simulink model "disturbance_est"  (R2020b)
settings: Solver=FixedStepAuto  StartTime=0.0  StopTime=10  FixedStep=0.01  RelTol=1e-3
values from neighbouring files (symbols this model uses):
  G = -J_RH*(M_M*L/2+M*l)*(J_RH+N^2*J_m+j)*g    (= -0.22537747671)    [aaaaaaaaaaaaaaaaaaaaaaaaa.m]    (also in disturb_estimation.m = -0.0465293382657; full_obs2.m = -0.0465293382657; fuulll_feedback.m = -0.0465293382657; reduced_observre_2.m = -0.0465293382657)
  H = -N*K_m*J_RH    (= -0.00759948)    [aaaaaaaaaaaaaaaaaaaaaaaaa.m]    (also in disturb_estimation.m = -0.00486576; full_obs2.m = -0.00486576; fuulll_feedback.m = -0.00486576; reduced_observre_2.m = -0.00486576)
  k1 = K(1)    [disturb_estimation.m]    (also in full_obs2.m; fuulll_feedback.m; reduced_observre_2.m)
  k2 = K(2)    [disturb_estimation.m]    (also in full_obs2.m; fuulll_feedback.m; reduced_observre_2.m)
  k3 = K(3)    [disturb_estimation.m]    (also in full_obs2.m; fuulll_feedback.m; reduced_observre_2.m)
  k4 = K(4)    [disturb_estimation.m]    (also in full_obs2.m; fuulll_feedback.m; reduced_observre_2.m)
  k5 = K(5)    [disturb_estimation.m]    (also in full_obs2.m; fuulll_feedback.m; reduced_observre_2.m)
  K_m = 0.0109    [aaaaaaaaaaaaaaaaaaaaaaaaa.m]    (also in disturb_estimation.m; full_obs2.m; fuulll_feedback.m; reduced_observre_2.m)
  l1 = L(1)    [disturb_estimation.m]    (also in full (2).m = 0.06; full_obs2.m)
  l2 = L(2)    [disturb_estimation.m]    (also in full (2).m = 0.6329; full_obs2.m)
  l3 = L(3)    [disturb_estimation.m]    (also in full (2).m = 0.3; full_obs2.m)
  l4 = L(4)    [disturb_estimation.m]    (also in full (2).m = 0.0875; full_obs2.m)
  l5 = L(5)    [disturb_estimation.m]    (also in full (2).m = 0.0254; full_obs2.m)
  l6 = 160    [disturb_estimation.m]    (also in full_obs2.m = 100)
  L_m = 0.145    [aaaaaaaaaaaaaaaaaaaaaaaaa.m]    (also in disturb_estimation.m; full_obs2.m; fuulll_feedback.m; reduced_observre_2.m)
  N = 14    [aaaaaaaaaaaaaaaaaaaaaaaaa.m]    (also in disturb_estimation.m = 3; full (2).m = -1.06605676; full_obs2.m = 3; fuulll_feedback.m = 3)
  R_m = 1.6    [aaaaaaaaaaaaaaaaaaaaaaaaa.m]    (also in disturb_estimation.m; full_obs2.m; fuulll_feedback.m; reduced_observre_2.m)
  T = (M_M*L/2+M*l)*(J_RH+N^2*J_m+j)*g    (= 4.52565214276)    [aaaaaaaaaaaaaaaaaaaaaaaaa.m]    (also in disturb_estimation.m = 0.312697165764; full (2).m = [T1;T2;T3;T4;T5;T6;T7]; full_obs2.m = 0.312697165764; fuulll_feedback.m = 0.312697165764)
  W = (J_M+M*l^2)*(J_RH+N^2*J_m+j)-(J_RH)^2    (= 0.0397505665657)    [aaaaaaaaaaaaaaaaaaaaaaaaa.m]    (also in disturb_estimation.m = -0.0192235420783; full (2).m = blkdiag(W_1,W_2,W_3,W_4,W_5,W_6,W_7); full_obs2.m = -0.0192235420783; fuulll_feedback.m = -0.0192235420783)
  Z = (J_M+M*l^2)*(J_RH+N^2*J_m+j)^2-J_RH^2*(J_RH+N^2*J_m+j)    (= 0.251295170273)    [aaaaaaaaaaaaaaaaaaaaaaaaa.m]    (also in disturb_estimation.m = -0.00839686182665; full_obs2.m = -0.00839686182665; fuulll_feedback.m = -0.00839686182665; reduced_observre_2.m = -0.00839686182665)
libraries: simulink x1
settings Model: Creator=A family  LastModifiedBy=A family

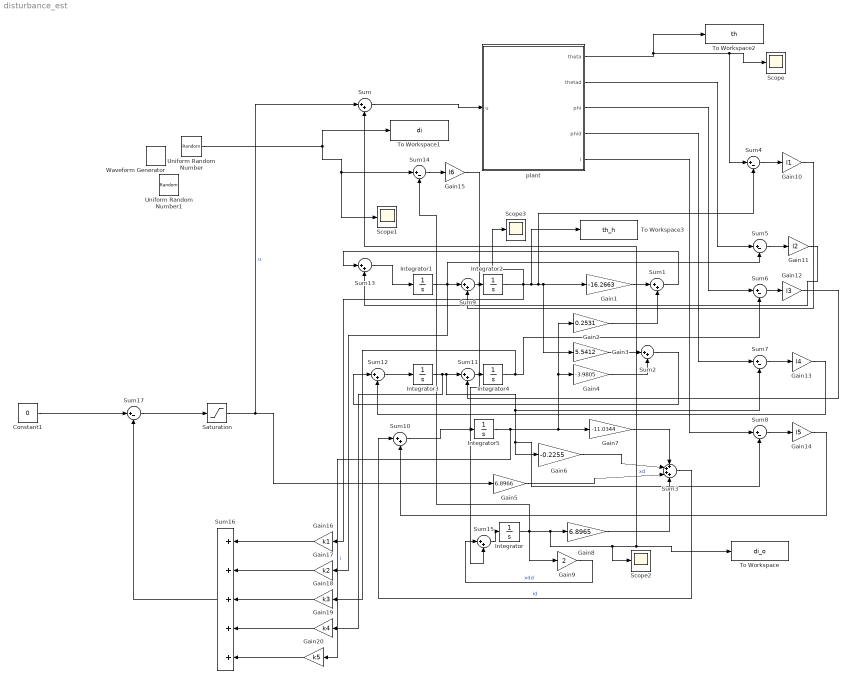
== system disturbance_est ==
  Constant1 : Constant  Value=0
  Gain1 : Gain  Gain=-16.2663
  Gain10 : Gain  Gain=l1
  Gain11 : Gain  Gain=l2
  Gain12 : Gain  Gain=l3
  Gain13 : Gain  Gain=l4
  Gain14 : Gain  Gain=l5
  Gain15 : Gain  Gain=l6
  Gain16 : Gain  Gain=k1
  Gain17 : Gain  Gain=k2
  Gain18 : Gain  Gain=k3
  Gain19 : Gain  Gain=k4
  Gain2 : Gain  Gain=0.2531
  Gain20 : Gain  Gain=k5
  Gain3 : Gain  Gain=5.5412
  Gain4 : Gain  Gain=-3.9805
  Gain5 : Gain  Gain=6.8966
  Gain6 : Gain  Gain=-0.2255
  Gain7 : Gain  Gain=-11.0344
  Gain8 : Gain  Gain=6.8965
  Gain9 : Gain  Gain=2
  Integrator{,1..5} (6 alike) : Integrator
  Saturation : Saturate  UpperLimit=6  LowerLimit=-6
  Scope{,1..3} (4 alike) : Scope
  Sum{,1..2,9..13,15} (9 alike) : Sum  Inputs=|++
  Sum{4..8,14,17} (7 alike) : Sum  Inputs=|+-
  Sum16 : Sum  Inputs=+++++
  Sum3 : Sum  Inputs=++++
  To Workspace : ToWorkspace  VariableName=di_o  SampleTime=-1
  To Workspace1 : ToWorkspace  VariableName=di  SampleTime=-1
  To Workspace2 : ToWorkspace  VariableName=th  SampleTime=-1
  To Workspace3 : ToWorkspace  VariableName=th_h  SampleTime=-1
  Uniform Random Number : UniformRandomNumber  Minimum=-4  Maximum=4  SampleTime=0.01
  Uniform Random Number1 : UniformRandomNumber  Minimum=-4  Maximum=4  SampleTime=0.01
  Waveform Generator : simulink/Sources/Waveform Generator  OutMin=[]  OutMax=[]  OutDataTypeStr=double  SelectedSignal=1  BlockNames=MultiportSwitch_e3df3653d217406  SampleTime=0.1
  plant : Subsystem
  wires:
  Gain1/1 -> Sum1/1
  Gain2/1 -> Sum1/2
  Sum1/1 -> Sum13/1
  Integrator5/1 -> Gain20/1, Gain2/1, Gain4/1, Gain7/1  "i"
  Integrator3/1 -> Gain19/1, Sum11/1, Sum7/2, Sum8/2, Gain6/1
  Gain3/1 -> Sum2/1
  Gain4/1 -> Sum2/2
  Sum2/1 -> Sum12/1
  Sum3/1 -> Sum10/1  "id"
  Saturation/1 -> Gain5/1, Sum/1  "u"
  Gain9/1 -> Sum15/1  "xdd"
  Integrator/1 -> Sum14/2, Gain9/1, Sum/2, To Workspace/1, Scope2/1, Gain8/1  "xd"
  Gain7/1 -> Sum3/1
  Gain8/1 -> Sum3/4
  Gain6/1 -> Sum3/2
  Gain5/1 -> Sum3/3
  Uniform Random Number/1 -> Scope1/1, Sum14/1, To Workspace1/1
  Sum4/1 -> Gain10/1
  plant/2(thetad) -> Sum5/1
  Sum5/1 -> Gain11/1
  plant/3(phi) -> Sum6/1
  Integrator4/1 -> Gain18/1, Sum6/2
  Sum6/1 -> Gain12/1
  plant/4(phid) -> Sum7/1
  Sum7/1 -> Gain13/1
  plant/5(i) -> Sum8/1
  Sum8/1 -> Gain14/1
  Integrator1/1 -> Gain17/1, Sum5/2, Sum9/1
  Sum9/1 -> Integrator2/1
  Gain10/1 -> Sum9/2
  Gain11/1 -> Sum13/2
  Integrator2/1 -> Gain1/1, Gain3/1, Sum4/2, To Workspace3/1, Gain16/1, Scope3/1
  Gain12/1 -> Sum11/2
  Sum11/1 -> Integrator4/1
  Gain13/1 -> Sum12/2
  Sum12/1 -> Integrator3/1
  Sum13/1 -> Integrator1/1
  Gain14/1 -> Sum10/2
  Sum10/1 -> Integrator5/1
  Sum14/1 -> Gain15/1
  Gain15/1 -> Sum15/2
  Sum15/1 -> Integrator/1
  plant/1(theta) -> To Workspace2/1, Scope/1, Sum4/1
  Gain18/1 -> Sum16/3
  Gain16/1 -> Sum16/1
  Gain20/1 -> Sum16/5
  Gain19/1 -> Sum16/4
  Gain17/1 -> Sum16/2
  Sum16/1 -> Sum17/2
  Constant1/1 -> Sum17/1
  Sum17/1 -> Saturation/1
  Sum/1 -> plant/1(u)

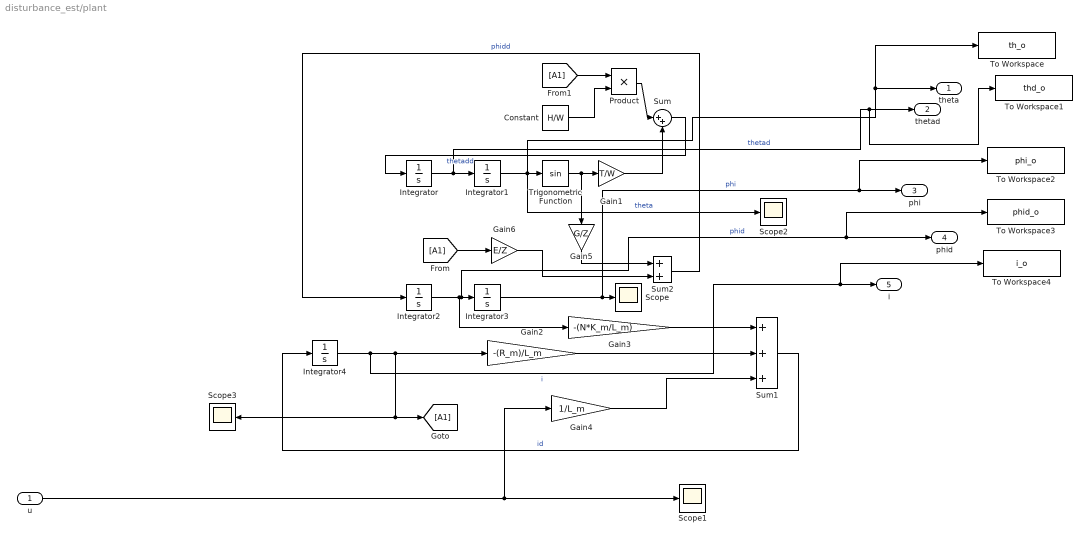
== system disturbance_est/plant ==
  u : Inport
  Constant : Constant  Value=H/W
  Gain1 : Gain  Gain=T/W
  Gain2 : Gain  Gain=-(R_m)/L_m
  Gain3 : Gain  Gain=-(N*K_m/L_m)
  Gain4 : Gain  Gain=1/L_m
  Gain5 : Gain  Gain=G/Z
  Gain6 : Gain  Gain=E/Z
  Integrator{,2..4} (4 alike) : Integrator
  Integrator1 : Integrator  InitialCondition=20*pi/180
  Product : Product
  Scope{,1..3} (4 alike) : Scope
  Sum : Sum  Inputs=|++
  Sum1 : Sum  Inputs=+++
  Sum2 : Sum
  To Workspace : ToWorkspace  VariableName=th_o  SampleTime=-1
  To Workspace1 : ToWorkspace  VariableName=thd_o  SampleTime=-1
  To Workspace2 : ToWorkspace  VariableName=phi_o  SampleTime=-1
  To Workspace3 : ToWorkspace  VariableName=phid_o  SampleTime=-1
  To Workspace4 : ToWorkspace  VariableName=i_o  SampleTime=-1
  Trigonometric Function : Trigonometry
  theta : Outport
  thetad : Outport  Port=2
  phi : Outport  Port=3
  phid : Outport  Port=4
  i : Outport  Port=5
  wires:
  Integrator/1 -> To Workspace1/1, thetad/1, Integrator1/1  "thetad"
  Integrator2/1 -> To Workspace3/1, phid/1, Integrator3/1, Gain3/1  "phid"
  Integrator4/1 -> Gain2/1, Scope3/1, [A1], To Workspace4/1, i/1  "i"
  Gain5/1 -> Sum2/1
  u/1 -> Scope1/1, Gain4/1
  Product/1 -> Sum/1
  Sum2/1 -> Integrator2/1  "phidd"
  Integrator1/1 -> To Workspace/1, theta/1, Scope2/1, Trigonometric Function/1  "theta"
  Gain4/1 -> Sum1/3
  Integrator3/1 -> To Workspace2/1, phi/1, Scope/1  "phi"
  [A1] -> Gain6/1
  Gain6/1 -> Sum2/2
  [A1] -> Product/1
  Constant/1 -> Product/2
  Gain1/1 -> Sum/2
  Trigonometric Function/1 -> Gain5/1, Gain1/1
  Gain3/1 -> Sum1/1
  Gain2/1 -> Sum1/2
  Sum1/1 -> Integrator4/1  "id"
  Sum/1 -> Integrator/1  "thetadd"
